simulink model "hydra_model"  (R2014b)
settings: configuration reference "SimulationConfig" (kept outside this file)
undefined symbols (not defined in the file or in its folder): gcbh, rmidispblock
libraries: NXTFcns x2, ControllersFcns x2
PreSaveFcn:
  | % Creates new data dictionary based on template.
  | 
  | projRoot = ETRoboconUtilities.getCheckoutRoot;
  | dictName = [bdroot 'Data.sldd'];
  | 
  | source = fullfile(projRoot,'templates','RobotTemplateData.sldd');
  | dest = fullfile(projRoot,'data_dictionaries',dictName);
  | 
  | if ~exist(dest) && ~isequal(bdroot,'RobotTemplate')
  |   copyfile(source,dest);
  |   disp(['Created new dictionary ' dictName ' in the data_dictionaries folder.']);
  |   set_param(bdroot,'DataDictionary', dictName);
  | end
Description:
  | ET Robocon 2014 robot template model.
  | 
  | Author:  Sebastian Castro
settings Model: DataDictionary=hydra_modelData.sldd  ExtModeTrigDuration=2  Creator=mbiesiad  LastModifiedBy=pkaniara

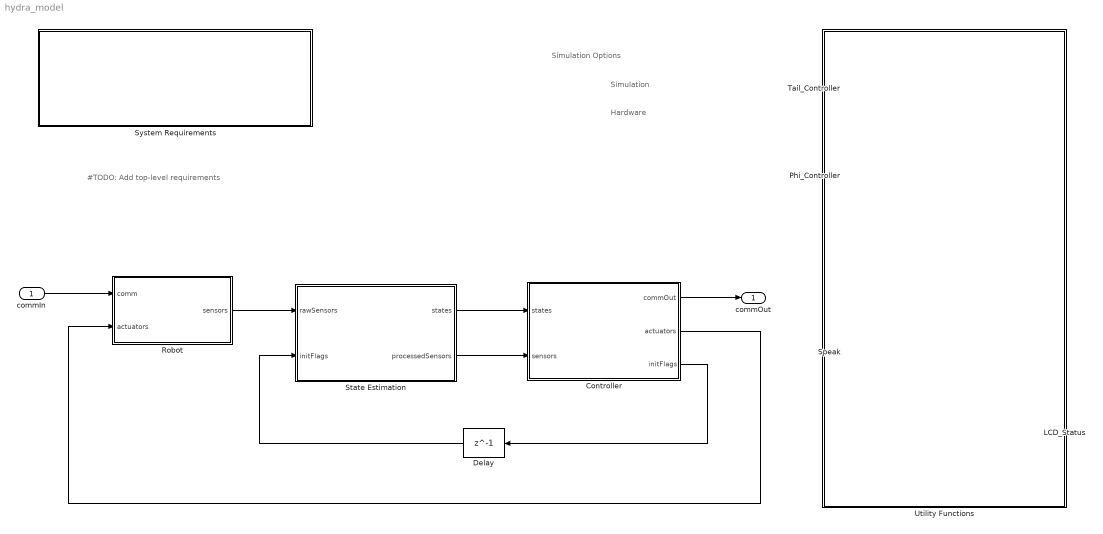
== system hydra_model ==
  note: #TODO:
      | Add top-level requirements
  note: Simulation Options
  note: Simulation
  note: Hardware
  commIn : Inport
  Controller : Stateflow chart  TreatAsAtomicUnit=on
  Delay : Delay  DelayLength=1
      settings: AttributesFormatString=Removes algebraic loop
  LCD_Status : NXTFcns/LCD_Status
  Phi_Controller : ControllersFcns/Phi_Controller
  Robot : Subsystem  Variant=on  VariantControl=Variant1
  Speak : NXTFcns/Speak
  State Estimation : Subsystem
  System Requirements : Subsystem  LoadFcn=rmidispblock('load',gcbh)  mask(System Requirements){id=SystemReq, title=System Requirements}
      mask prompts: title "Block Title"
      mask help: Lists the requirements for the current model.
      mask init:
      | id = 'SystemReq';
      | [w,h] = rmidispblock('display',gcbh);
      settings: CopyFcn=rmidispblock('create',gcbh)  DeleteFcn=rmidispblock('delete',gcbh)  ModelCloseFcn=rmidispblock('close',gcbh)  PreSaveFcn=rmidispblock('close',gcbh)  PostSaveFcn=rmidispblock('open',gcbh)  OpenFcn=rmidispblock('open',gcbh)  MoveFcn=rmidispblock('move',gcbh)
      mask Help: helpview(fullfile(docroot,'toolbox','slvnv','slvnv.map'),'systemrequirements')
      mask Display:
      | text(326/2,113-4,rmidispblock('title',gcbh),'horizontalAlignment','center','verticalAlignment','top')
      | text(w/2,h/2,'<No Requirements in System>','horizontalAlignment','center','verticalAlignment','top')
  Tail_Controller : ControllersFcns/Tail_Controller
  Utility Functions : Subsystem
  commOut : Outport
  wires:
  State Estimation/2(processedSensors) -> Controller/2(sensors)
  Robot/1(sensors) -> State Estimation/1(rawSensors)
  Controller/3(initFlags) -> Delay/1
  State Estimation/1(states) -> Controller/1(states)
  Delay/1 -> State Estimation/2(initFlags)
  Controller/2(actuators) -> Robot/2(actuators)
  Controller/1(commOut) -> commOut/1
  commIn/1 -> Robot/1(comm)

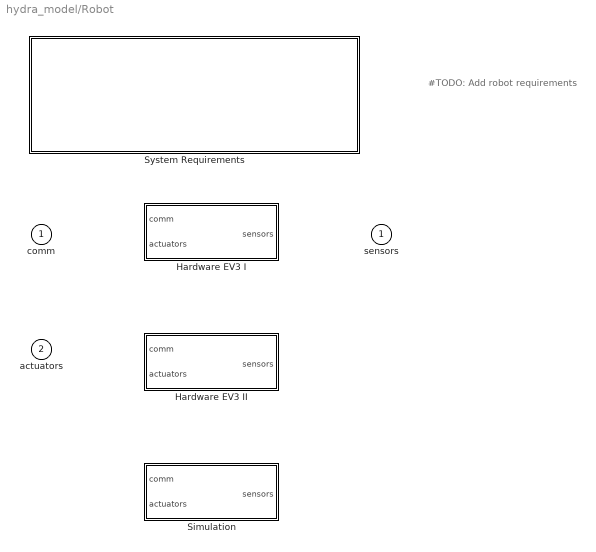
== system hydra_model/Robot ==
  note: #TODO:
      | Add robot requirements
  comm : Inport
  actuators : Inport  Port=2
  Hardware EV3 I : Subsystem  VariantControl=HardwareVar
  Hardware EV3 II : Subsystem  VariantControl=HardwareVar
  Simulation : Subsystem  VariantControl=SimulationVar
  System Requirements : Subsystem  LoadFcn=rmidispblock('load',gcbh)  VariantControl=Variant  mask(System Requirements){id=SystemReq, title=System Requirements}
      mask prompts: title "Block Title"
      mask help: Lists the requirements for the current model.
      mask init:
      | id = 'SystemReq';
      | [w,h] = rmidispblock('display',gcbh);
      settings: CopyFcn=rmidispblock('create',gcbh)  DeleteFcn=rmidispblock('delete',gcbh)  ModelCloseFcn=rmidispblock('close',gcbh)  PreSaveFcn=rmidispblock('close',gcbh)  PostSaveFcn=rmidispblock('open',gcbh)  OpenFcn=rmidispblock('open',gcbh)  MoveFcn=rmidispblock('move',gcbh)
      mask Help: helpview(fullfile(docroot,'toolbox','slvnv','slvnv.map'),'systemrequirements')
      mask Display:
      | text(326/2,113-4,rmidispblock('title',gcbh),'horizontalAlignment','center','verticalAlignment','top')
      | text(w/2,h/2,'<No Requirements in System>','horizontalAlignment','center','verticalAlignment','top')
  sensors : Outport

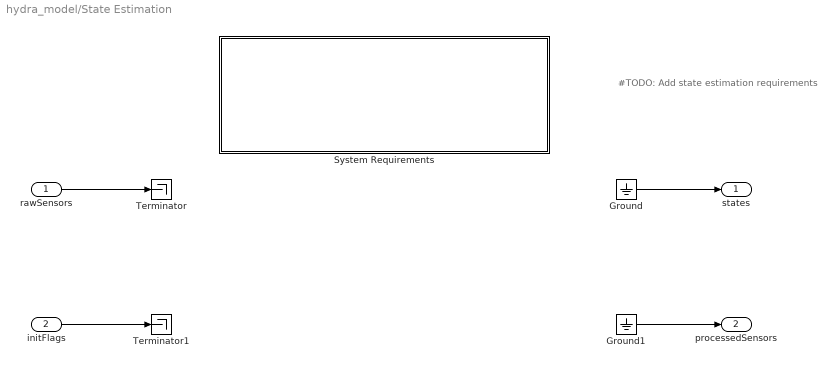
== system hydra_model/State Estimation ==
  note: #TODO:
      | Add state estimation requirements
  rawSensors : Inport
  initFlags : Inport  Port=2
  Ground : Ground
  Ground1 : Ground
  System Requirements : Subsystem  LoadFcn=rmidispblock('load',gcbh)  mask(System Requirements){id=SystemReq, title=System Requirements}
      mask prompts: title "Block Title"
      mask help: Lists the requirements for the current model.
      mask init:
      | id = 'SystemReq';
      | [w,h] = rmidispblock('display',gcbh);
      settings: CopyFcn=rmidispblock('create',gcbh)  DeleteFcn=rmidispblock('delete',gcbh)  ModelCloseFcn=rmidispblock('close',gcbh)  PreSaveFcn=rmidispblock('close',gcbh)  PostSaveFcn=rmidispblock('open',gcbh)  OpenFcn=rmidispblock('open',gcbh)  MoveFcn=rmidispblock('move',gcbh)
      mask Help: helpview(fullfile(docroot,'toolbox','slvnv','slvnv.map'),'systemrequirements')
      mask Display:
      | text(326/2,113-4,rmidispblock('title',gcbh),'horizontalAlignment','center','verticalAlignment','top')
      | text(w/2,h/2,'<No Requirements in System>','horizontalAlignment','center','verticalAlignment','top')
  Terminator : Terminator
  Terminator1 : Terminator
  states : Outport
  processedSensors : Outport  Port=2
  wires:
  initFlags/1 -> Terminator1/1
  Ground/1 -> states/1
  Ground1/1 -> processedSensors/1
  rawSensors/1 -> Terminator/1

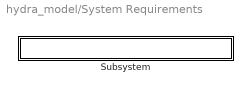
== system hydra_model/System Requirements ==
  Subsystem : Subsystem  mask{label=0, index=1}
      mask init:
      | label = rmidispblock('label',index);
      settings: OpenFcn=rmidispblock('openReq',gcbh);
      mask Display: text(0,0,label,'horizontalAlignment','left','verticalAlignment','bottom')

== system hydra_model/Utility Functions ==

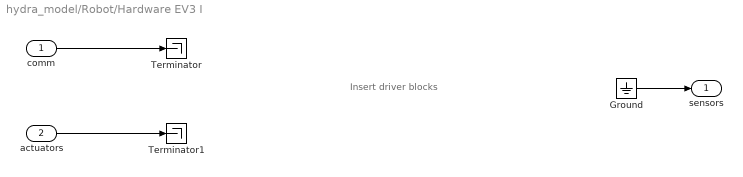
== system hydra_model/Robot/Hardware EV3 I ==
  note: Insert driver blocks
  comm : Inport
  actuators : Inport  Port=2
  Ground : Ground
  Terminator : Terminator
  Terminator1 : Terminator
  sensors : Outport
  wires:
  Ground/1 -> sensors/1
  actuators/1 -> Terminator1/1
  comm/1 -> Terminator/1

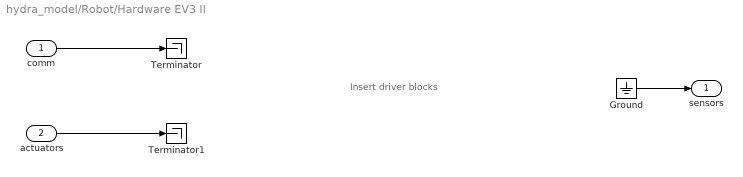
== system hydra_model/Robot/Hardware EV3 II ==
  note: Insert driver blocks
  comm : Inport
  actuators : Inport  Port=2
  Ground : Ground
  Terminator : Terminator
  Terminator1 : Terminator
  sensors : Outport
  wires:
  comm/1 -> Terminator/1
  actuators/1 -> Terminator1/1
  Ground/1 -> sensors/1

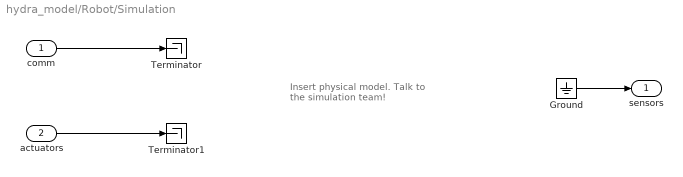
== system hydra_model/Robot/Simulation ==
  note: Insert physical model.
      | Talk to the simulation team!
  comm : Inport
  actuators : Inport  Port=2
  Ground : Ground
  Terminator : Terminator
  Terminator1 : Terminator
  sensors : Outport
  wires:
  Ground/1 -> sensors/1
  actuators/1 -> Terminator1/1
  comm/1 -> Terminator/1

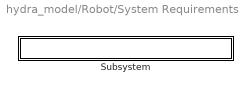
== system hydra_model/Robot/System Requirements ==
  Subsystem : Subsystem  mask{label=0, index=1}
      mask init:
      | label = rmidispblock('label',index);
      settings: OpenFcn=rmidispblock('openReq',gcbh);
      mask Display: text(0,0,label,'horizontalAlignment','left','verticalAlignment','bottom')

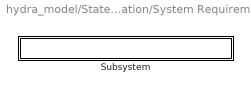
== system hydra_model/State Estimation/System Requirements ==
  Subsystem : Subsystem  mask{label=0, index=1}
      mask init:
      | label = rmidispblock('label',index);
      settings: OpenFcn=rmidispblock('openReq',gcbh);
      mask Display: text(0,0,label,'horizontalAlignment','left','verticalAlignment','bottom')

== system hydra_model/System Requirements/Subsystem ==

== system hydra_model/Robot/System Requirements/Subsystem ==

== system hydra_model/State Estimation/System Requirements/Subsystem ==

== stateflow chart hydra_model/Controller ==
  state Tail Balance
    % Add control logic here.
  note: #TODO
      | Add requirements to Stateflow objects
      | by right-clicking and selecting the
      | Requirements Traceability option.
  (default) -> Tail Balance
  data: commOut output single size=1; actuators output Bus: PWM_bus size=1; states input Bus: States_Bus size=1; sensors input Bus: Sensors_Bus size=1; initFlags output Bus: Init_Bus size=1
